simulink model "IsaqueMIC2esp32"  (R2023a)
settings: Solver=VariableStepAuto  StartTime=0.0  StopTime=16  RelTol=1e-3
libraries: instrumentlib x8, cstblocks x4, simulink x1
settings Model: Creator=Aluno - LPR 6  LastModifiedBy=Aluno - LPR 6

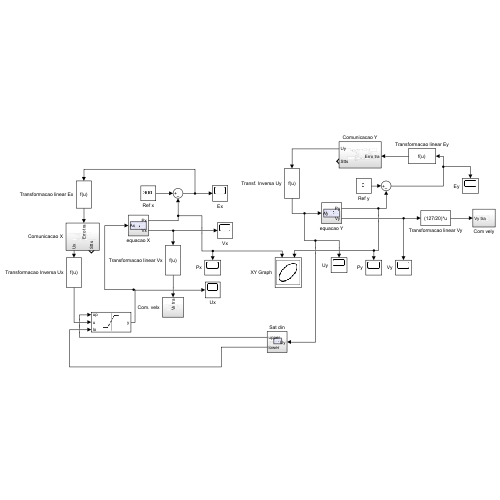
[thumbnail: Simulink's stored preview of the top-level diagram]
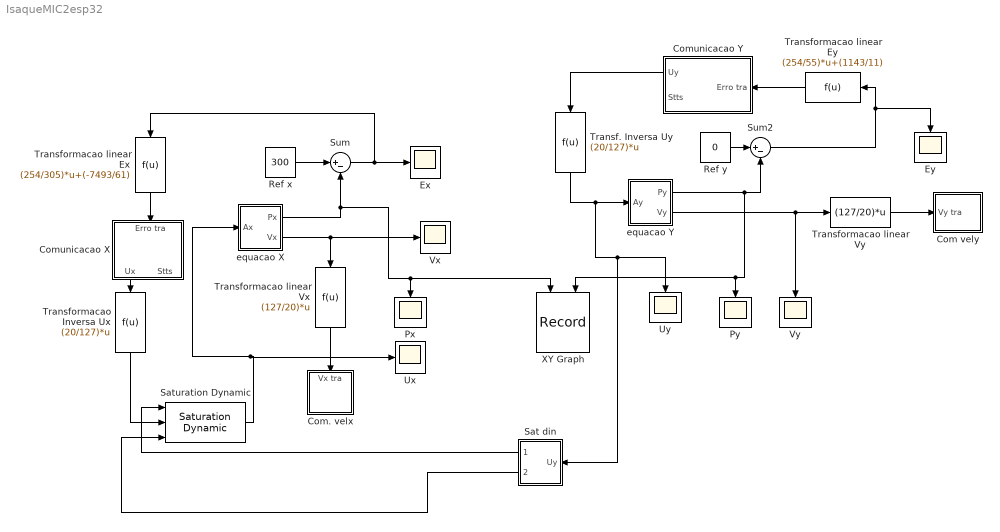
== system IsaqueMIC2esp32 ==
  Com vely : Subsystem
  Com. velx : Subsystem
  Comunicacao X : Subsystem
  Comunicacao Y : Subsystem
  Ex : Scope
  Ey : Scope
  Px : Scope
  Py : Scope
  Ref x : Constant  Value=300
  Ref y : Constant  Value=0
  Sat din : Subsystem
  Saturation Dynamic : simulink/Discontinuities/Saturation Dynamic  OutMin=[]  OutMax=[]  OutDataTypeStr=Inherit: Same as second input  OutDataType=fixdt(1, 16)  OutScaling=2^-10  DoSatur=off
  Sum : Sum  Inputs=|+-
  Sum2 : Sum  Inputs=|+-
  Transf. Inversa Uy : Fcn  Expr=(20/127)*u
  Transformacao Inversa Ux : Fcn  Expr=(20/127)*u
  Transformacao linear Ex : Fcn  Expr=(254/305)*u+(-7493/61)
  Transformacao linear Ey : Fcn  Expr=(254/55)*u+(1143/11)
  Transformacao linear Vx : Fcn  Expr=(127/20)*u
  Transformacao linear Vy : Fcn  Expr=(127/20)*u
  Ux : Scope
  Uy : Scope
  Vx : Scope
  Vy : Scope
  XY Graph : Record  FileSettingsInternal="{\"entries\":[{\"content\":{\"excelSettings\":{\"content\":{},\"type\":\"Streamout.ExcelSettings\"}},\"type\":\"Streamout.FileSettingStorage\",\"uuid\":\"256d3897-134c-4c5b-92f3-51154ac2da76\"}],\"packageUris\":[\"http://schema.mathworks.com/mf0/streamout_blocks/R2020a\"],\"version\":\"1.0\"}"  Layout=[1 1]  SignalsInternal="{\"entries\":[{\"content\":{\"signals\":[{\"content\":{\"blockPath\":[\"IsaqueMIC2esp32/XY Graph\"],\"dimensions\":[1],\"domain\":\"IsaqueMIC2esp32/XY Graph\",\"lineColor\":\"#a2142f\",\"plots\":[1],\"port\":1,\"sid\":[\"\"],\"signalID\":196559,\"signalName\":\"equacao X:1\"},\"type\":\"RecordBlkView.Signal\",\"uuid\":\"2905abe8-010f-41a8-b1fd-e10e9030ab0a\"},{\"content\":{\"blockPath\":[\"IsaqueMIC2esp32/XY Graph\"],\"dimensions\":[1],\"domain\":\"IsaqueMIC2esp32/XY Graph\",\"lineColor\":\"#139fff\",\"plots\":[1],\"port\":2,\"sid\":[\"\"],\"signalID\":196563,\"signalName\":\"equacao Y:1\"},\"type\":\"RecordBlkView.Signal\",\"uuid\":\"c9dc01c2-55c2-4149-9981-6b48f50ea08d\"}]},\"type\":\"RecordBlkView.InputSignals\",\"uuid\":\"54ce684d-0e54-4f82-ab55-41bbc2f158ea\"}],\"packageUris\":[\"http://schema.mathworks.com/mf0/streamout_blocks/R2020a\"],\"version\":\"1.0\"}"  VisualizationBindings="{\"xyplotplugin\":{\"info\":[{\"series\":[{\"bindingParametersList\":[{\"parameter\":\"X-Axis\",\"signalID\":196559,\"signalName\":\"equacao X:1\"},{\"parameter\":\"Y-Axis\",\"signalID\":196563,\"signalName\":\"equacao Y:1\"}],\"seriesID\":58891}],\"subplotID\":1}]}}"  CompatibilityTag=XY
  equacao X : Subsystem
  equacao Y : Subsystem
  wires:
  Sum/1 -> Transformacao linear Ex/1, Ex/1
  equacao X/2(Vx) -> Vx/1, Transformacao linear Vx/1
  Ref y/1 -> Sum2/1
  equacao X/1(Px) -> XY Graph/1, Px/1, Sum/2
  equacao Y/2(Vy) -> Transformacao linear Vy/1, Vy/1
  Ref x/1 -> Sum/1
  equacao Y/1(Py) -> Sum2/2, XY Graph/2, Py/1
  Transformacao linear Ex/1 -> Comunicacao X/1(Erro tra)
  Comunicacao X/1(Ux) -> Transformacao Inversa Ux/1
  Transformacao linear Vx/1 -> Com. velx/1(Vx tra)
  Transformacao linear Ey/1 -> Comunicacao Y/1(Erro tra)
  Transformacao linear Vy/1 -> Com vely/1(Vy tra)
  Comunicacao Y/1(Uy) -> Transf. Inversa Uy/1
  Transf. Inversa Uy/1 -> equacao Y/1(Ay), Sat din/1(Uy), Uy/1
  Sum2/1 -> Ey/1, Transformacao linear Ey/1
  Sat din/1(upper) -> Saturation Dynamic/1
  Sat din/2(lower) -> Saturation Dynamic/3
  Transformacao Inversa Ux/1 -> Saturation Dynamic/2
  Saturation Dynamic/1 -> Ux/1, equacao X/1(Ax)

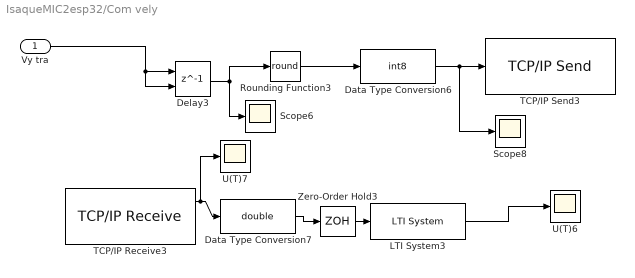
== system IsaqueMIC2esp32/Com vely ==
  Vy tra : Inport
  Data Type Conversion6 : DataTypeConversion  OutDataTypeStr=int8  SaturateOnIntegerOverflow=off  RndMeth=Floor
  Data Type Conversion7 : DataTypeConversion  OutDataTypeStr=double  SaturateOnIntegerOverflow=off  RndMeth=Floor
  Delay3 : Delay  DelayLength=1  InitialConditionSource=Input port  InitialCondition=0
      settings: InputPortMap=u0,p4
  LTI System3 : cstblocks/LTI System  sys=tf(1,[0.05 1])  IC=[]
  Rounding Function3 : Rounding  Operator=round
  Scope6 : Scope
  Scope8 : Scope
  TCP/IP Receive3 : instrumentlib/TCP//IP Receive  Host=192.168.4.1  Port=5003  DataSize=[ 1, 1 ]  DataType=int8  ASCIIFormatting=%f  Terminator=CR  CustomTerminator=10  ByteOrder=big-endian  EnableBlockingMode=off  Timeout=10  SampleTime=0.0001  SimulateUsing=Interpreted execution
  TCP/IP Send3 : instrumentlib/TCP//IP Send  Host=192.168.4.1  Port=5003  ByteOrder=big-endian  EnableBlockingMode=off  Timeout=10  TransferDelay=on  SimulateUsing=Interpreted execution
  U(T)6 : Scope
  U(T)7 : Scope
  Zero-Order Hold3 : ZeroOrderHold  SampleTime=0.0001
  wires:
  TCP/IP Receive3/1 -> U(T)7/1, Data Type Conversion7/1
  Data Type Conversion7/1 -> Zero-Order Hold3/1
  Data Type Conversion6/1 -> Scope8/1, TCP/IP Send3/1
  Delay3/1 -> Rounding Function3/1, Scope6/1
  Zero-Order Hold3/1 -> LTI System3/1
  Vy tra/1 -> Delay3/2, Delay3/1
  LTI System3/1 -> U(T)6/1
  Rounding Function3/1 -> Data Type Conversion6/1

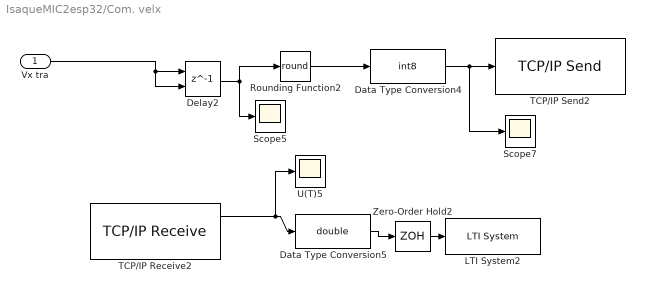
== system IsaqueMIC2esp32/Com. velx ==
  Vx tra : Inport
  Data Type Conversion4 : DataTypeConversion  OutDataTypeStr=int8  SaturateOnIntegerOverflow=off  RndMeth=Floor
  Data Type Conversion5 : DataTypeConversion  OutDataTypeStr=double  SaturateOnIntegerOverflow=off  RndMeth=Floor
  Delay2 : Delay  DelayLength=1  InitialConditionSource=Input port  InitialCondition=0
      settings: InputPortMap=u0,p4
  LTI System2 : cstblocks/LTI System  sys=tf(1,[0.05 1])  IC=[]
  Rounding Function2 : Rounding  Operator=round
  Scope5 : Scope
  Scope7 : Scope
  TCP/IP Receive2 : instrumentlib/TCP//IP Receive  Host=192.168.4.1  Port=5002  DataSize=[ 1, 1 ]  DataType=int8  ASCIIFormatting=%f  Terminator=CR  CustomTerminator=10  ByteOrder=big-endian  EnableBlockingMode=off  Timeout=10  SampleTime=0.0001  SimulateUsing=Interpreted execution
  TCP/IP Send2 : instrumentlib/TCP//IP Send  Host=192.168.4.1  Port=5002  ByteOrder=big-endian  EnableBlockingMode=off  Timeout=10  TransferDelay=on  SimulateUsing=Interpreted execution
  U(T)5 : Scope
  Zero-Order Hold2 : ZeroOrderHold  SampleTime=0.0001
  wires:
  Rounding Function2/1 -> Data Type Conversion4/1
  Vx tra/1 -> Delay2/2, Delay2/1
  Zero-Order Hold2/1 -> LTI System2/1
  TCP/IP Receive2/1 -> U(T)5/1, Data Type Conversion5/1
  Data Type Conversion4/1 -> Scope7/1, TCP/IP Send2/1
  Data Type Conversion5/1 -> Zero-Order Hold2/1
  Delay2/1 -> Rounding Function2/1, Scope5/1

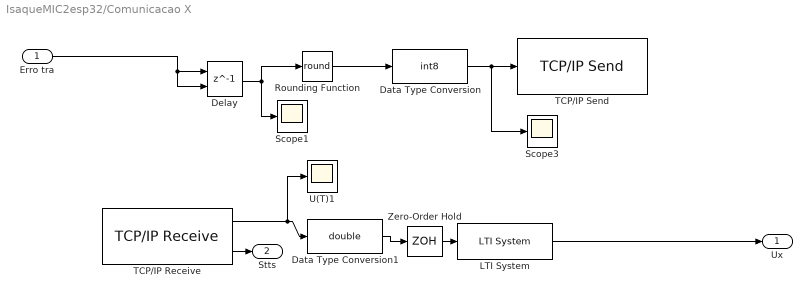
== system IsaqueMIC2esp32/Comunicacao X ==
  Erro tra : Inport
  Data Type Conversion : DataTypeConversion  OutDataTypeStr=int8  SaturateOnIntegerOverflow=off  RndMeth=Floor
  Data Type Conversion1 : DataTypeConversion  OutDataTypeStr=double  SaturateOnIntegerOverflow=off  RndMeth=Floor
  Delay : Delay  DelayLength=1  InitialConditionSource=Input port  InitialCondition=0
      settings: InputPortMap=u0,p4
  LTI System : cstblocks/LTI System  sys=tf(1,[0.05 1])  IC=[]
  Rounding Function : Rounding  Operator=round
  Scope1 : Scope
  Scope3 : Scope
  TCP/IP Receive : instrumentlib/TCP//IP Receive  Host=192.168.4.1  Port=5000  DataSize=[ 1, 1 ]  DataType=int8  ASCIIFormatting=%f  Terminator=CR  CustomTerminator=10  ByteOrder=big-endian  EnableBlockingMode=off  Timeout=10  SampleTime=0.0001  SimulateUsing=Interpreted execution
  TCP/IP Send : instrumentlib/TCP//IP Send  Host=192.168.4.1  Port=5000  ByteOrder=big-endian  EnableBlockingMode=off  Timeout=10  TransferDelay=on  SimulateUsing=Interpreted execution
  U(T)1 : Scope
  Zero-Order Hold : ZeroOrderHold  SampleTime=0.0001
  Ux : Outport
  Stts : Outport  Port=2
  wires:
  Zero-Order Hold/1 -> LTI System/1
  Data Type Conversion/1 -> Scope3/1, TCP/IP Send/1
  Data Type Conversion1/1 -> Zero-Order Hold/1
  Erro tra/1 -> Delay/2, Delay/1
  TCP/IP Receive/1 -> U(T)1/1, Data Type Conversion1/1
  Delay/1 -> Rounding Function/1, Scope1/1
  Rounding Function/1 -> Data Type Conversion/1
  TCP/IP Receive/2 -> Stts/1
  LTI System/1 -> Ux/1

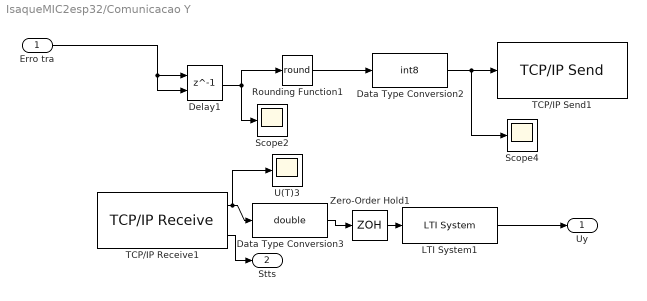
== system IsaqueMIC2esp32/Comunicacao Y ==
  Erro tra : Inport
  Data Type Conversion2 : DataTypeConversion  OutDataTypeStr=int8  SaturateOnIntegerOverflow=off  RndMeth=Floor
  Data Type Conversion3 : DataTypeConversion  OutDataTypeStr=double  SaturateOnIntegerOverflow=off  RndMeth=Floor
  Delay1 : Delay  DelayLength=1  InitialConditionSource=Input port  InitialCondition=0
      settings: InputPortMap=u0,p4
  LTI System1 : cstblocks/LTI System  sys=tf(1,[0.05 1])  IC=[]
  Rounding Function1 : Rounding  Operator=round
  Scope2 : Scope
  Scope4 : Scope
  TCP/IP Receive1 : instrumentlib/TCP//IP Receive  Host=192.168.4.1  Port=5001  DataSize=[ 1, 1 ]  DataType=int8  ASCIIFormatting=%f  Terminator=CR  CustomTerminator=10  ByteOrder=big-endian  EnableBlockingMode=off  Timeout=10  SampleTime=0.0001  SimulateUsing=Interpreted execution
  TCP/IP Send1 : instrumentlib/TCP//IP Send  Host=192.168.4.1  Port=5001  ByteOrder=big-endian  EnableBlockingMode=off  Timeout=10  TransferDelay=on  SimulateUsing=Interpreted execution
  U(T)3 : Scope
  Zero-Order Hold1 : ZeroOrderHold  SampleTime=0.0001
  Uy : Outport
  Stts : Outport  Port=2
  wires:
  Data Type Conversion2/1 -> Scope4/1, TCP/IP Send1/1
  TCP/IP Receive1/1 -> U(T)3/1, Data Type Conversion3/1
  Rounding Function1/1 -> Data Type Conversion2/1
  TCP/IP Receive1/2 -> Stts/1
  Delay1/1 -> Rounding Function1/1, Scope2/1
  Erro tra/1 -> Delay1/2, Delay1/1
  Zero-Order Hold1/1 -> LTI System1/1
  Data Type Conversion3/1 -> Zero-Order Hold1/1
  LTI System1/1 -> Uy/1

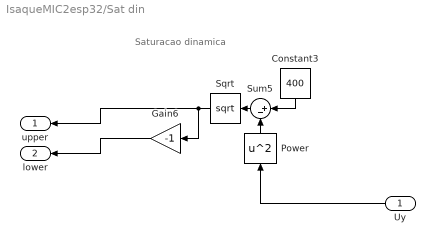
== system IsaqueMIC2esp32/Sat din ==
  note: Saturacao dinamica
  Uy : Inport
  Constant3 : Constant  Value=400
  Gain6 : Gain  Gain=-1
  Power : Math  Operator=square
  Sqrt : Sqrt
  Sum5 : Sum  Inputs=|+-
  upper : Outport
  lower : Outport  Port=2
  wires:
  Uy/1 -> Power/1
  Gain6/1 -> lower/1
  Sqrt/1 -> upper/1, Gain6/1
  Sum5/1 -> Sqrt/1
  Constant3/1 -> Sum5/1
  Power/1 -> Sum5/2

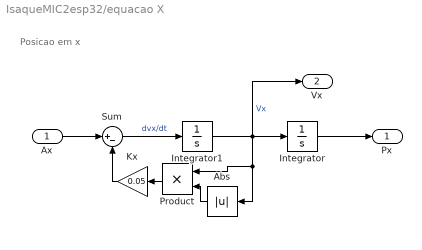
== system IsaqueMIC2esp32/equacao X ==
  note: Posicao em x
  Ax : Inport
  Abs : Abs  SaturateOnIntegerOverflow=off
  Integrator : Integrator  InitialCondition=45
  Integrator1 : Integrator  InitialCondition=18.6
  Kx : Gain  Gain=0.05
  Product : Product
  Sum : Sum  Inputs=|+-
  Px : Outport
  Vx : Outport  Port=2
  wires:
  Integrator1/1 -> Product/1, Abs/1, Vx/1, Integrator/1  "Vx"
  Ax/1 -> Sum/1
  Integrator/1 -> Px/1
  Kx/1 -> Sum/2
  Sum/1 -> Integrator1/1  "dvx/dt"
  Product/1 -> Kx/1
  Abs/1 -> Product/2

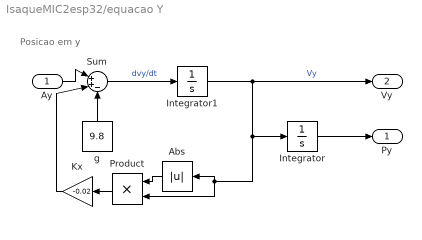
== system IsaqueMIC2esp32/equacao Y ==
  note: Posicao em y
  Ay : Inport
  Abs : Abs  SaturateOnIntegerOverflow=off
  Integrator : Integrator  InitialCondition=40
  Integrator1 : Integrator  InitialCondition=-14.74
  Kx : Gain  Gain=-0.02
  Product : Product
  Sum : Sum  Inputs=|++-
  g : Constant  Value=9.8
  Py : Outport
  Vy : Outport  Port=2
  wires:
  Integrator1/1 -> Vy/1, Product/2, Abs/1, Integrator/1  "Vy"
  Ay/1 -> Sum/1
  Kx/1 -> Sum/2
  g/1 -> Sum/3
  Sum/1 -> Integrator1/1  "dvy/dt"
  Integrator/1 -> Py/1
  Product/1 -> Kx/1
  Abs/1 -> Product/1
